simulink model "DC_twin"  (R2021a)
settings: Solver=VariableStepAuto  StartTime=0.0  StopTime=10  MaxStep=1e-4  RelTol=1e-3
values from neighbouring files (symbols this model uses):
  gr = 1024    [DC_twin_parameters.m]
  Imax = 2*Inom    (= 3.58)    [DC_twin_parameters.m]
  J = 2.56e4    (= 25600)    [Apollo_LM_design_discrete_observer.m]    (also in Apollo_LM_design_observer.m; Apollo_LM_observer_feedback.m; Apollo_LM_state_feedback.m; DC_twin_parameters.m = 22.8675707733)
  k = Vnom / w_no_load    (= 0.0309706916287)    [DC_twin_parameters.m]    (also in partial_exam_facit.m = 2)
  k_cc = 25    [DC_twin_parameters.m]
  L = place(A, B, pd)    [Apollo_LM_design_discrete_observer.m]    (also in Apollo_LM_design_observer.m = L_a; Apollo_LM_observer_feedback.m = [l1, l2, l3]; Apollo_LM_state_feedback.m = [l1, l2, l3]; DC_twin_parameters.m = 0.000268)
  R = 1.75    [DC_twin_parameters.m]
  tau_i_cc = 0.1    [DC_twin_parameters.m]
  Vmax = 1.5*Vnom    (= 54)    [DC_twin_parameters.m]
libraries: pid_lib x2
settings Model: Creator=kjartan  LastModifiedBy=kjartan

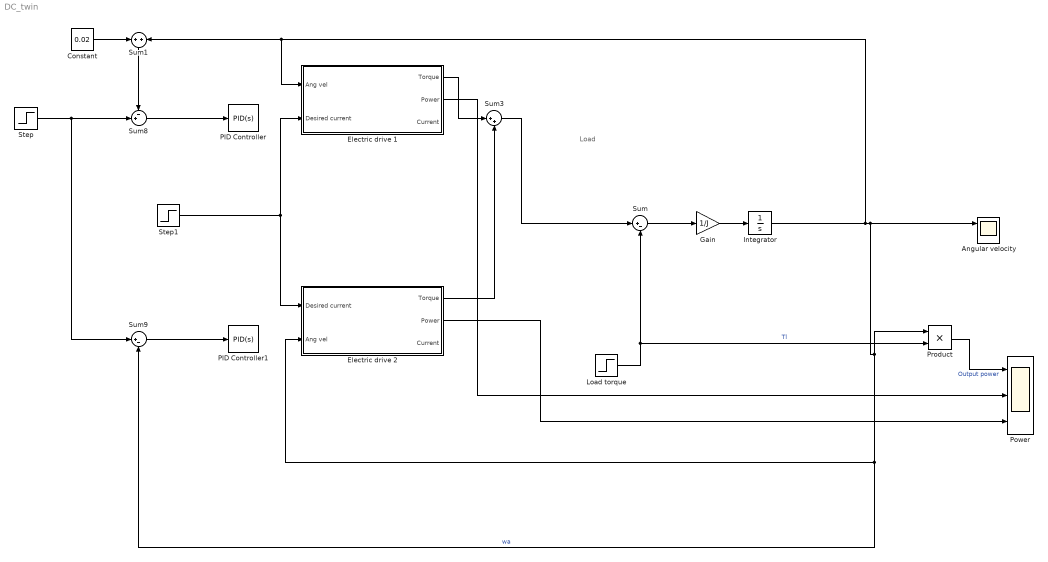
== system DC_twin ==
  note: Load
  Angular velocity : Scope  NumInputPorts=3
  Constant : Constant  Value=0.02
  Electric drive 1 : Subsystem
  Electric drive 2 : Subsystem
  Gain : Gain  Gain=1/J
  Integrator : Integrator
  Load torque : Step  After=10  SampleTime=0
  PID Controller : pid_lib/PID Controller  Controller=PID  Form=Ideal  TimeDomain=Continuous-time  UseExternalTs=off  SampleTime=-1  IntegratorMethod=Forward Euler  FilterMethod=Forward Euler  ControllerParametersSource=internal  P=1  I=1  D=0  UseFilter=on  N=100  TunerSelectOption=Transfer Function Based (PID Tuner App)  InitialConditionSource=internal  InitialConditionForIntegrator=0  InitialConditionForFilter=0  DifferentiatorICPrevScaledInput=0  ExternalReset=none  TrackingMode=off  Kt=1  LimitOutput=off  SatLimitsSource=internal  UpperSaturationLimit=inf  LowerSaturationLimit=-inf  LinearizeAsGain=on  AntiWindupMode=none  Kb=1  POutMin=[]  POutMax=[]  IOutMin=[]  IOutMax=[]  DOutMin=[]  DOutMax=[]  NOutMin=[]  NOutMax=[]  SumOutMin=[]  SumOutMax=[]  SaturationOutMin=[]  SaturationOutMax=[]  PParamMin=[]  PParamMax=[]  IParamMin=[]  IParamMax=[]  DParamMin=[]  DParamMax=[]  NParamMin=[]  NParamMax=[]  KbParamMin=[]  KbParamMax=[]  KtParamMin=[]  KtParamMax=[]  KbOutMin=[]  KbOutMax=[]  KtOutMin=[]  KtOutMax=[]  IntegratorOutMin=[]  IntegratorOutMax=[]  FilterOutMin=[]  FilterOutMax=[]  SumI1OutMin=[]  SumI1OutMax=[]  SumI2OutMin=[]  SumI2OutMax=[]  SumI3OutMin=[]  SumI3OutMax=[]  SumI4OutMin=[]  SumI4OutMax=[]  SumDOutMin=[]  SumDOutMax=[]  DifferentiatorOutMin=[]  DifferentiatorOutMax=[]  FilterDiffOutCoefMin=[]  FilterDiffOutCoefMax=[]  ReciprocalOutMin=[]  ReciprocalOutMax=[]  SumDenOutMin=[]  SumDenOutMax=[]  SumNumOutMin=[]  SumNumOutMax=[]  DivideOutMin=[]  DivideOutMax=[]  UdiffTsProdOutMin=[]  UdiffTsProdOutMax=[]  NTsProdOutMin=[]  NTsProdOutMax=[]  UintegralTsProdOutMin=[]  UintegralTsProdOutMax=[]  UngainTsProdOutMin=[]  UngainTsProdOutMax=[]  IntegratorContinuousStateAttributes=''  IntegratorStateMustResolveToSignalObject=off  IntegratorRTWStateStorageClass=Auto  FilterContinuousStateAttributes=''  FilterStateMustResolveToSignalObject=off  FilterRTWStateStorageClass=Auto  ParallelPVariant=Passthrough  IdealPVariant=InternalParameters  IVariant=InternalParameters  DVariant=InternalParameters  IntegratorVariant=Continuous  SatVariant=Disabled  AWVariant=Passthrough  PCopyVariant=Disabled  TRVariant=Disabled  FdbkBlocksVariant=Forward  IdealPFdbkVariant=Disabled  SatFdbkVariant=Disabled  DerivativeFilterVariant=ContFilter  NVariant=InternalParameters  NCopyVariant=Disabled  FilterICVariant=InternalICsFilter  IntegratorICVariant=InternalICs  ExternalResetVariant=Disabled  TRSumVariant=Passthrough  SumFdbkVariant=Disabled  SumVariant=Sum_PID  TsampFilterVariant=InternalTs  TsampNgainVariant=Passthrough  TsampIntegralVariant=Passthrough  ExternalSaturationOutDataTypeStr=Inherit: Same as second input
  PID Controller1 : pid_lib/PID Controller  Controller=PID  Form=Parallel  TimeDomain=Continuous-time  UseExternalTs=off  SampleTime=-1  IntegratorMethod=Forward Euler  FilterMethod=Forward Euler  ControllerParametersSource=internal  P=1  I=1  D=0  UseFilter=on  N=100  TunerSelectOption=Transfer Function Based (PID Tuner App)  InitialConditionSource=internal  InitialConditionForIntegrator=0  InitialConditionForFilter=0  DifferentiatorICPrevScaledInput=0  ExternalReset=none  TrackingMode=off  Kt=1  LimitOutput=off  SatLimitsSource=internal  UpperSaturationLimit=inf  LowerSaturationLimit=-inf  LinearizeAsGain=on  AntiWindupMode=none  Kb=1  POutMin=[]  POutMax=[]  IOutMin=[]  IOutMax=[]  DOutMin=[]  DOutMax=[]  NOutMin=[]  NOutMax=[]  SumOutMin=[]  SumOutMax=[]  SaturationOutMin=[]  SaturationOutMax=[]  PParamMin=[]  PParamMax=[]  IParamMin=[]  IParamMax=[]  DParamMin=[]  DParamMax=[]  NParamMin=[]  NParamMax=[]  KbParamMin=[]  KbParamMax=[]  KtParamMin=[]  KtParamMax=[]  KbOutMin=[]  KbOutMax=[]  KtOutMin=[]  KtOutMax=[]  IntegratorOutMin=[]  IntegratorOutMax=[]  FilterOutMin=[]  FilterOutMax=[]  SumI1OutMin=[]  SumI1OutMax=[]  SumI2OutMin=[]  SumI2OutMax=[]  SumI3OutMin=[]  SumI3OutMax=[]  SumI4OutMin=[]  SumI4OutMax=[]  SumDOutMin=[]  SumDOutMax=[]  DifferentiatorOutMin=[]  DifferentiatorOutMax=[]  FilterDiffOutCoefMin=[]  FilterDiffOutCoefMax=[]  ReciprocalOutMin=[]  ReciprocalOutMax=[]  SumDenOutMin=[]  SumDenOutMax=[]  SumNumOutMin=[]  SumNumOutMax=[]  DivideOutMin=[]  DivideOutMax=[]  UdiffTsProdOutMin=[]  UdiffTsProdOutMax=[]  NTsProdOutMin=[]  NTsProdOutMax=[]  UintegralTsProdOutMin=[]  UintegralTsProdOutMax=[]  UngainTsProdOutMin=[]  UngainTsProdOutMax=[]  IntegratorContinuousStateAttributes=''  IntegratorStateMustResolveToSignalObject=off  IntegratorRTWStateStorageClass=Auto  FilterContinuousStateAttributes=''  FilterStateMustResolveToSignalObject=off  FilterRTWStateStorageClass=Auto  ParallelPVariant=InternalParameters  IdealPVariant=Disabled  IVariant=InternalParameters  DVariant=InternalParameters  IntegratorVariant=Continuous  SatVariant=Disabled  AWVariant=Passthrough  PCopyVariant=Disabled  TRVariant=Disabled  FdbkBlocksVariant=Forward  IdealPFdbkVariant=Disabled  SatFdbkVariant=Disabled  DerivativeFilterVariant=ContFilter  NVariant=InternalParameters  NCopyVariant=Disabled  FilterICVariant=InternalICsFilter  IntegratorICVariant=InternalICs  ExternalResetVariant=Disabled  TRSumVariant=Passthrough  SumFdbkVariant=Disabled  SumVariant=Sum_PID  TsampFilterVariant=InternalTs  TsampNgainVariant=Passthrough  TsampIntegralVariant=Passthrough  ExternalSaturationOutDataTypeStr=Inherit: Same as second input
  Power : Scope  NumInputPorts=3
  Product : Product
  Step : Step  Time=0  SampleTime=0
  Step1 : Step  Time=0  SampleTime=0
  Sum : Sum  Inputs=|+-
  Sum1 : Sum  Inputs=+|+
  Sum3 : Sum  Inputs=|++
  Sum8 : Sum  Inputs=-+|
  Sum9 : Sum  Inputs=|+-
  wires:
  Sum/1 -> Gain/1
  Gain/1 -> Integrator/1
  Load torque/1 -> Product/2, Sum/2  "Tl"
  Integrator/1 -> Electric drive 1/1(Ang vel), Sum1/2, Electric drive 2/2(Ang vel), Sum9/2, Product/1, Angular velocity/1  "wa"
  Sum3/1 -> Sum/1
  Product/1 -> Power/1  "Output power"
  Step/1 -> Sum9/1, Sum8/2
  Sum8/1 -> PID Controller/1
  Sum9/1 -> PID Controller1/1
  Electric drive 1/1(Torque) -> Sum3/1
  Electric drive 2/1(Torque) -> Sum3/2
  Electric drive 2/2(Power) -> Power/3
  Electric drive 1/2(Power) -> Power/2
  Sum1/1 -> Sum8/1
  Constant/1 -> Sum1/1
  Step1/1 -> Electric drive 2/1(Desired current), Electric drive 1/2(Desired current)

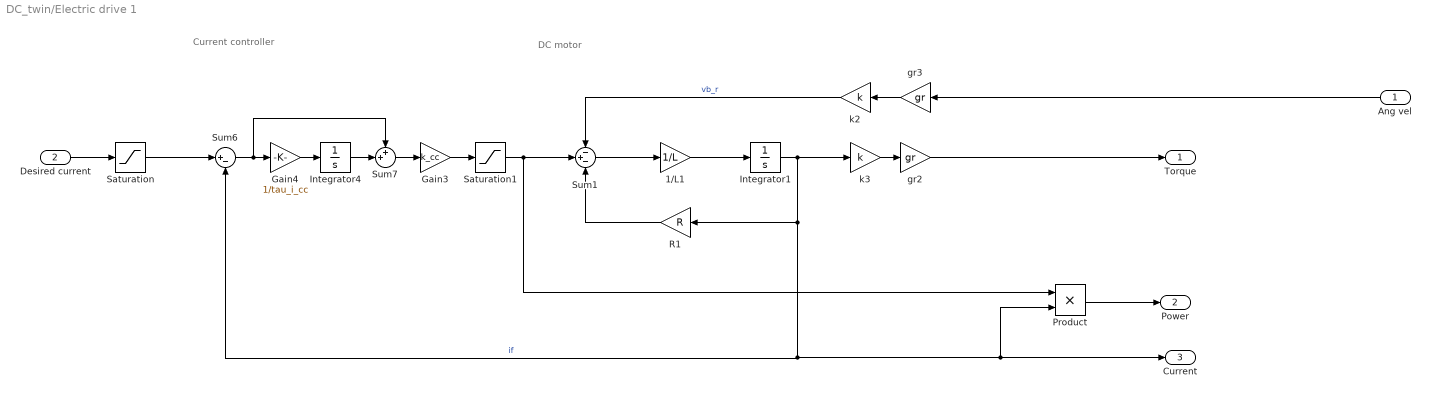
== system DC_twin/Electric drive 1 ==
  note: Current controller
  note: DC motor
  Ang vel : Inport
  Desired current : Inport  Port=2
  1/L1 : Gain  Gain=1/L
  Gain3 : Gain  Gain=k_cc
  Gain4 : Gain  Gain=1/tau_i_cc
  Integrator1 : Integrator
  Integrator4 : Integrator
  Product : Product
  R1 : Gain  Gain=R
  Saturation : Saturate  UpperLimit=Imax  LowerLimit=-Imax
  Saturation1 : Saturate  UpperLimit=Vmax  LowerLimit=-Vmax
  Sum1 : Sum  Inputs=-+-
  Sum6 : Sum  Inputs=|+-
  Sum7 : Sum  Inputs=++|
  gr2 : Gain  Gain=gr
  gr3 : Gain  Gain=gr
  k2 : Gain  Gain=k
  k3 : Gain  Gain=k
  Torque : Outport
  Power : Outport  Port=2
  Current : Outport  Port=3
  wires:
  Saturation/1 -> Sum6/1
  Sum1/1 -> 1/L1/1
  Saturation1/1 -> Product/1, Sum1/2
  R1/1 -> Sum1/3
  gr2/1 -> Torque/1
  Integrator1/1 -> k3/1, R1/1, Product/2, Current/1, Sum6/2  "if"
  Gain4/1 -> Integrator4/1
  Ang vel/1 -> gr3/1
  Desired current/1 -> Saturation/1
  Sum6/1 -> Gain4/1, Sum7/1
  gr3/1 -> k2/1
  k2/1 -> Sum1/1  "vb_r"
  Integrator4/1 -> Sum7/2
  Gain3/1 -> Saturation1/1
  1/L1/1 -> Integrator1/1
  Sum7/1 -> Gain3/1
  k3/1 -> gr2/1
  Product/1 -> Power/1

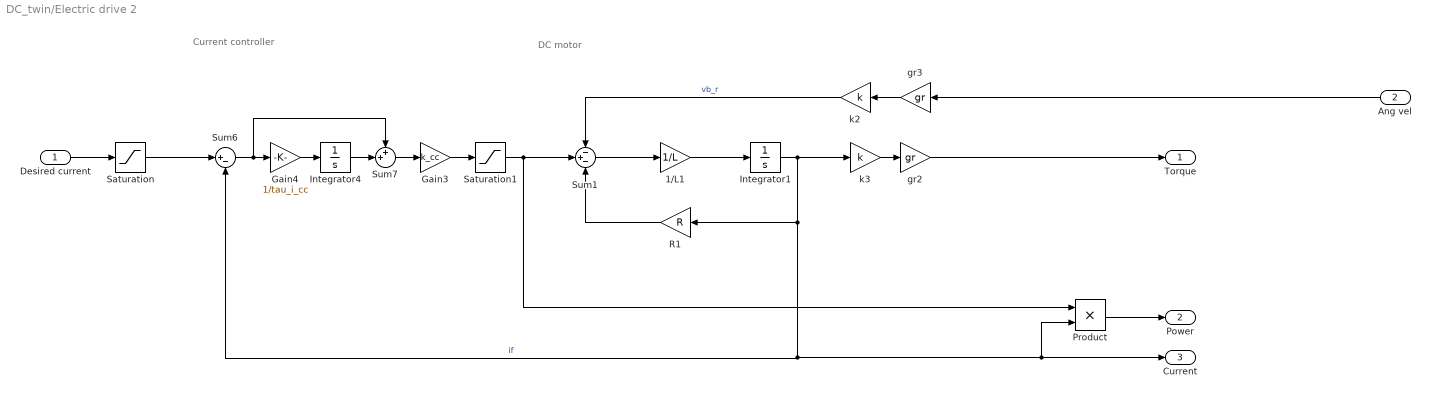
== system DC_twin/Electric drive 2 ==
  note: DC motor
  note: Current controller
  Desired current : Inport
  Ang vel : Inport  Port=2
  1/L1 : Gain  Gain=1/L
  Gain3 : Gain  Gain=k_cc
  Gain4 : Gain  Gain=1/tau_i_cc
  Integrator1 : Integrator
  Integrator4 : Integrator
  Product : Product
  R1 : Gain  Gain=R
  Saturation : Saturate  UpperLimit=Imax  LowerLimit=-Imax
  Saturation1 : Saturate  UpperLimit=Vmax  LowerLimit=-Vmax
  Sum1 : Sum  Inputs=-+-
  Sum6 : Sum  Inputs=|+-
  Sum7 : Sum  Inputs=++|
  gr2 : Gain  Gain=gr
  gr3 : Gain  Gain=gr
  k2 : Gain  Gain=k
  k3 : Gain  Gain=k
  Torque : Outport
  Power : Outport  Port=2
  Current : Outport  Port=3
  wires:
  k3/1 -> gr2/1
  Sum7/1 -> Gain3/1
  1/L1/1 -> Integrator1/1
  Gain3/1 -> Saturation1/1
  Integrator4/1 -> Sum7/2
  k2/1 -> Sum1/1  "vb_r"
  gr3/1 -> k2/1
  Sum6/1 -> Sum7/1, Gain4/1
  Desired current/1 -> Saturation/1
  Ang vel/1 -> gr3/1
  Gain4/1 -> Integrator4/1
  Integrator1/1 -> Sum6/2, Product/2, Current/1, R1/1, k3/1  "if"
  gr2/1 -> Torque/1
  R1/1 -> Sum1/3
  Saturation1/1 -> Product/1, Sum1/2
  Sum1/1 -> 1/L1/1
  Saturation/1 -> Sum6/1
  Product/1 -> Power/1
